simulink model "PTC_MBDS_RSFlipFlop_Sample"  (R2013a)
settings: Solver=FixedStepDiscrete  StartTime=0.0  StopTime=100  FixedStep=Auto  RelTol=1e-3
undefined symbols (not defined in the file): sigbuilder_block
libraries: simulink_extras x1, PTC_MBDS_LIB x1
settings Model: Creator=uidl7367  LastModifiedBy=sundeep.tuteja
settings DataIOCC: SignalLoggingSaveFormat=ModelDataLogs
settings OptimizationCC: ExpressionDepthLimit=2147483647  InitFltsAndDblsToZero=on
settings DebuggingCC: SaveWithParameterizedLinksMsg=none  SignalResolutionControl=TryResolveAllWithWarning  SolverPrmCheckMsg=none  InheritedTsInSrcMsg=none  MultiTaskDSMMsg=warning  MultiTaskCondExecSysMsg=none  FcnCallInpInsideContextMsg=UseLocalSettings  StrictBusMsg=Warning
settings RTWCC: IncludeERTFirstTime=on
settings GRTTargetCC: TargetFcnLib=ansi_tfl_tmw.mat  CombineOutputUpdateFcns=off  GRTInterface=on

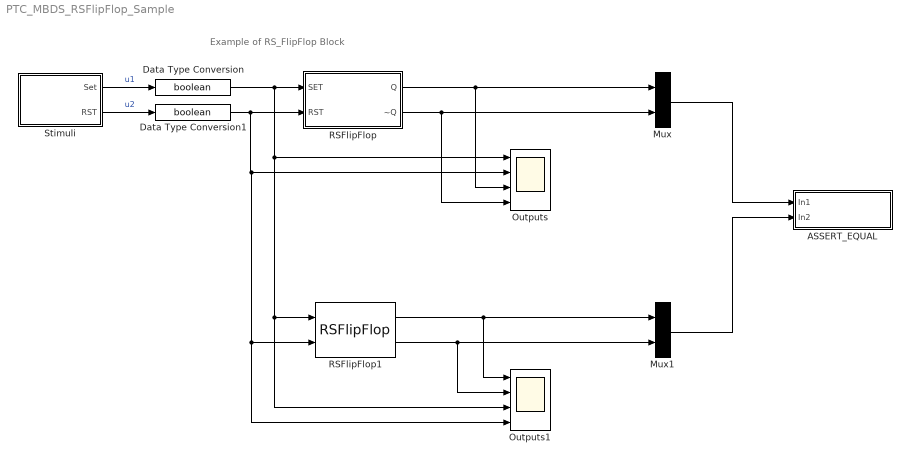
== system PTC_MBDS_RSFlipFlop_Sample ==
  note: Example of RS_FlipFlop Block
  ASSERT_EQUAL : Subsystem
  Data Type Conversion : DataTypeConversion  InitFcn=|  OutDataTypeStr=boolean  SaturateOnIntegerOverflow=on
      | try
      |    MBDS_BlockCallback('Update', gcb);
      | end
  Data Type Conversion1 : DataTypeConversion  InitFcn=|  OutDataTypeStr=boolean  SaturateOnIntegerOverflow=on
      | try
      |    MBDS_BlockCallback('Update', gcb);
      | end
  Mux : Mux  Inputs=2
  Mux1 : Mux  Inputs=2
  Outputs : Scope  NumInputPorts=4
      settings: TimeRange=100  YMin=0~0~0~0  YMax=1~1~1~1  SampleInput=on  SampleTime=1
  Outputs1 : Scope  NumInputPorts=4
      settings: TimeRange=100  YMin=0~0~0~0  YMax=1~1~1~1  SampleInput=on  SampleTime=1
  RSFlipFlop : Subsystem  InitFcn=|  mask(RSFlipFlop){MBDS_LibraryBlock=on, Q_Enabled=on, Not_Q_Enabled=on, MBDS_BlockVersion=05.40}
      | if(exist('MBDS_BlockCallback', 'file'))
      |    MBDS_BlockCallback('Update', gcb);
      | end
      mask prompts: MBDS_LibraryBlock "MBDS library block"; Q_Enabled "Show Q port"; Not_Q_Enabled "Show ~Q port"; MBDS_BlockVersion "Block version:"
      mask help: A flip flop. The reset input (RST) dominates the set input (SET).
      mask init:
      | if(exist('MBDS_BlockCallback', 'file'))
      |    MBDS_BlockCallback('Init', gcb);
      | else
      |    % Disable all mask parameters
      |    MaskEnables = get_param(gcb, 'MaskEnables');
      |    for k = [1:length(MaskEnables)]
      |       MaskEnables{k} = 'off';
      |    end
      |    if(~isequal(MaskEnables, get_param(gcb, 'MaskEnables')))
      |       set_param(gcb, 'MaskEnables', MaskEnables);
      |    end
      | end
      mask Help: eval(['open([workdir(''library_dir:''),''\Blockset\help\'',get_param(gcb,''MaskType''),''.html''])'])
      mask Callback Q_Enabled:
      | % Update mask parameter dialog
      | if(exist('MBDS_BlockCallback', 'file'))
      |    MBDS_BlockCallback('Q_Enabled', gcb);
      | end
      mask Callback Not_Q_Enabled:
      | % Update mask parameter dialog
      | if(exist('MBDS_BlockCallback', 'file'))
      |    MBDS_BlockCallback('Not_Q_Enabled', gcb);
      | end
      mask Display:
      | % Show icon or block text
      | if(exist('RSFlipFlop.tif', 'file'))
      |    image(imread('RSFlipFlop.tif','tif'), [0.295739348370927 0.17 0.378947368421053 0.66]);
      |    disp('')
      | else
      |    disp(sprintf('RS\nFlipFlop'));
      | end
      | 
      | % Display port labels
      | port_label('input', 1, 'SET');
      | port_label('input', 2, 'RST');
      | port_label('output', 1, 'Q');
      | port_label('output', 2, '~Q');
  RSFlipFlop1 : PTC_MBDS_LIB/MBDS Standard Library/Extended Operations/Memory Blocks/RSFlipFlop  Q_Enabled=on  Not_Q_Enabled=on  PTC_MBDS_BlockVersion=5.32  PTC_BlockType=PTC_MBDS_RSFlipFlop
  Stimuli : Subsystem  Tag=STV Subsys  LoadFcn=sigbuilder_block('load');  StartFcn=sigbuilder_block('start');  StopFcn=sigbuilder_block('stop');  ClipboardFcn=sigbuilder_block('clipboard');  mask(Sigbuilder block){}
      mask help: Sigbuilder GUI
      mask init:
      | if ~strcmp(get_param(bdroot(gcb),'SimulationStatus'),'stopped') tuvar = sigbuilder_block('maskInit'); end
      settings: CopyFcn=sigbuilder_block('copy');  DeleteFcn=sigbuilder_block('delete');  ModelCloseFcn=sigbuilder_block('modelClose');  PreSaveFcn=sigbuilder_block('preSave');  PauseFcn=sigbuilder_block('pause')  ContinueFcn=sigbuilder_block('continue')  NameChangeFcn=sigbuilder_block('namechange');  OpenFcn=sigbuilder_block('open',[1083 147.75 448.5 246 ]);  CloseFcn=sigbuilder_block('close');
      mask Display: plot(0,0,100,100,[10,10,40,40,10],[80,20,20,80,80],[40,10],[50,50], [40,27,10],[65,72,56],[40,25,25,10],[28,28,43,43]);
  wires:
  Stimuli/1(Set) -> Data Type Conversion/1  "u1"
  Stimuli/2(RST) -> Data Type Conversion1/1  "u2"
  RSFlipFlop/1(Q) -> Outputs/3, Mux/1
  RSFlipFlop/2(~Q) -> Outputs/4, Mux/2
  Data Type Conversion/1 -> RSFlipFlop/1(SET), RSFlipFlop1/1, Outputs1/3, Outputs/1
  Data Type Conversion1/1 -> RSFlipFlop/2(RST), RSFlipFlop1/2, Outputs1/4, Outputs/2
  RSFlipFlop1/2 -> Mux1/2, Outputs1/2
  RSFlipFlop1/1 -> Outputs1/1, Mux1/1
  Mux/1 -> ASSERT_EQUAL/1(In1)
  Mux1/1 -> ASSERT_EQUAL/2(In2)

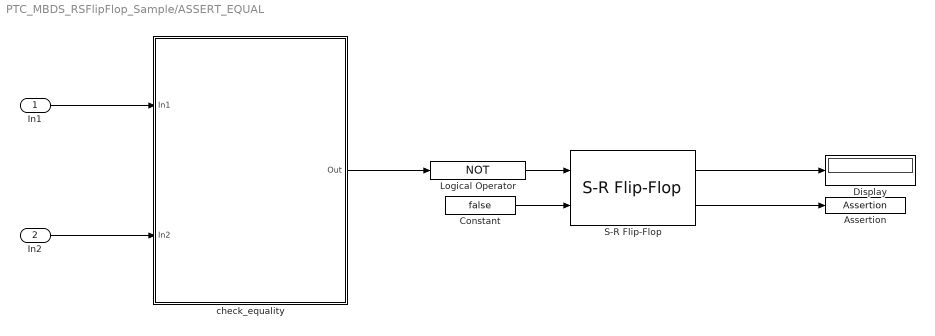
== system PTC_MBDS_RSFlipFlop_Sample/ASSERT_EQUAL ==
  In1 : Inport
  In2 : Inport  Port=2
  Assertion : Assertion
  Constant : Constant  Value=false
  Display : Display
  Logical Operator : Logic  Operator=NOT  AllPortsSameDT=off  OutDataTypeStr=boolean
  S-R Flip-Flop : simulink_extras/Flip Flops/S-R Flip-Flop  initial_condition=0
  check_equality : MATLAB Function  TreatAsAtomicUnit=on
  wires:
  S-R Flip-Flop/1 -> Display/1
  check_equality/1(Out) -> Logical Operator/1
  Constant/1 -> S-R Flip-Flop/2
  S-R Flip-Flop/2 -> Assertion/1
  In2/1 -> check_equality/2(In2)
  In1/1 -> check_equality/1(In1)
  Logical Operator/1 -> S-R Flip-Flop/1

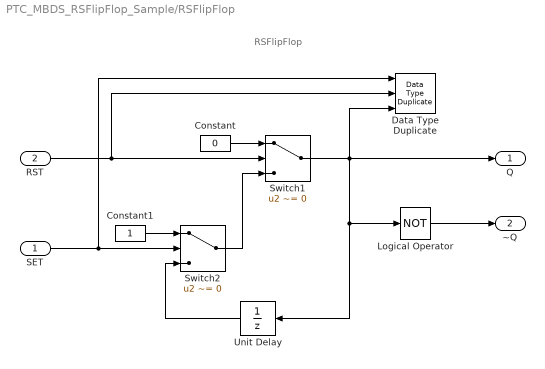
== system PTC_MBDS_RSFlipFlop_Sample/RSFlipFlop ==
  note: RSFlipFlop
  SET : Inport  OutDataTypeStr=boolean
  RST : Inport  Port=2  OutDataTypeStr=boolean
  Constant : Constant  Value=0  OutDataTypeStr=Inherit: Inherit via back propagation
  Constant1 : Constant  OutDataTypeStr=Inherit: Inherit via back propagation
  Data Type Duplicate : DataTypeDuplicate  NumInputPorts=3
  Logical Operator : Logic  Operator=NOT  AllPortsSameDT=off  OutDataTypeStr=boolean
  Switch1 : Switch  Criteria=u2 ~= 0  OutDataTypeStr=Inherit: Inherit via back propagation
  Switch2 : Switch  Criteria=u2 ~= 0  OutDataTypeStr=Inherit: Inherit via back propagation
  Unit Delay : UnitDelay  SampleTime=-1
  Q : Outport
  ~Q : Outport  Port=2
  wires:
  Switch1/1 -> Q/1, Data Type Duplicate/3, Unit Delay/1, Logical Operator/1
  Constant/1 -> Switch1/1
  RST/1 -> Data Type Duplicate/2, Switch1/2
  SET/1 -> Data Type Duplicate/1, Switch2/2
  Constant1/1 -> Switch2/1
  Switch2/1 -> Switch1/3
  Logical Operator/1 -> ~Q/1
  Unit Delay/1 -> Switch2/3

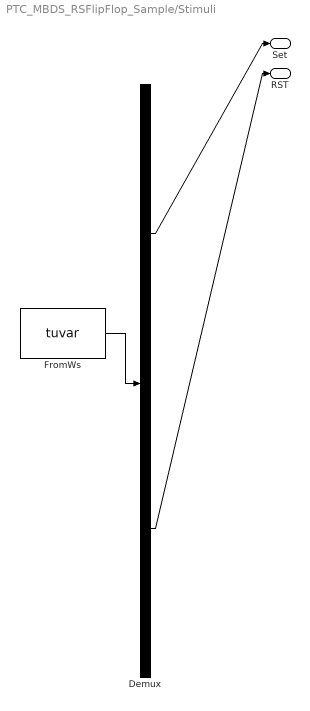
== system PTC_MBDS_RSFlipFlop_Sample/Stimuli ==
  Demux : Demux  Tag=STV Demux  Outputs=2
  FromWs : FromWorkspace  Tag=STV FromWs  VariableName=tuvar  SampleTime=1  OutputAfterFinalValue=Holding final value
      SigBuilderData=|
      | common.afterFinalStr = 'Hold final value'
      | common.sampleTime = 1
      | dataSet.timeRange = [0 10]
      | dataSet.name = 'test data'
      | sbobj.Groups.Name = 'test data'
      | sbobj.Groups.Signals(1).Name = 'Set'
      | sbobj.Groups.Signals(1).XData = [0 1 1 2 2 9 9 10]
      | sbobj.Groups.Signals(1).YData = [0 0 1 1 0 0 1 1]
      | sbobj.Groups.Signals(2).Name = 'RST'
      | sbobj.Groups.Signals(2).XData = [0 4 4 5 5 7 7 8 8 10]
      | sbobj.Groups.Signals(2).YData = [0 0 1 1 0 0 1 1 0 0]
  Set : Outport  Tag=STV Outport
  RST : Outport  Tag=STV Outport  Port=2
  wires:
  FromWs/1 -> Demux/1
  Demux/1 -> Set/1
  Demux/2 -> RST/1

== matlab function PTC_MBDS_RSFlipFlop_Sample/ASSERT_EQUAL/check_equality ==
  data: In1 input; Out output; In2 input
function Out = check_equality(In1, In2)
%#codegen

Out = isequaln(In1, In2);

end
